simulink model "wifiSwitch"  (R2019b)
settings: Solver=FixedStepAuto  StartTime=0.0  StopTime=inf  RelTol=1e-3  EnableMultiTasking=on
libraries: arduinolib x4
settings Model: SILPILModeSetting=veronly  ExtModeTrigDuration=2  Creator=lucciffer  LastModifiedBy=lucciffer
settings OptimizationCC: EnhancedBackFolding=on  PassReuseOutputArgsAs=Individual arguments  ZeroExternalMemoryAtStartup=off  ZeroInternalMemoryAtStartup=off  MaxStackSize=64  OptimizeBlockOrder=speed  DifferentSizesBufferReuse=on  OptimizationCustomize=off  EfficientTunableParamExpr=on
settings DebuggingCC: ParameterTunabilityLossMsg=error
settings HardwareCC: ProdBitPerInt=16  ProdBitPerPointer=16  ProdBitPerSizeT=16  ProdBitPerPtrDiffT=16  ProdLargestAtomicFloat=None  ProdWordSize=8  ProdHWDeviceType=Atmel->AVR  UseEmbeddedCoderFeatures=off
settings SFSimCC: MATLABDynamicMemAlloc=off
settings RTWCC: SystemTargetFile=ert.tlc  HardwareBoard=Arduino Mega 2560  TLCOptions=-aInlineSetEventsForThisBaseRateFcn=TLC_FALSE -aSuppressMultiTaskScheduler=TLC_FALSE -aRateBasedStepFcn=1  TemplateMakefile=ert_default_tmf  GenerateReport=on  Toolchain=Arduino AVR  BuildConfiguration=Faster Runs  IncludeHyperlinkInReport=on  LaunchReport=on  GenerateTraceInfo=on  GenerateTraceReport=on  GenerateTraceReportSl=on  GenerateTraceReportSf=on  GenerateTraceReportEml=on
settings CodeAppCC: ForceParamTrailComments=on  IgnoreCustomStorageClasses=off  OperatorAnnotations=on  SimulinkDataObjDesc=on  SFDataObjDesc=on  InsertBlockDesc=on
settings ERTTargetCC: SupportContinuousTime=on  SupportNonInlinedSFcns=on  SupportVariableSizeSignals=on  ExtModeStaticAllocSize=2048

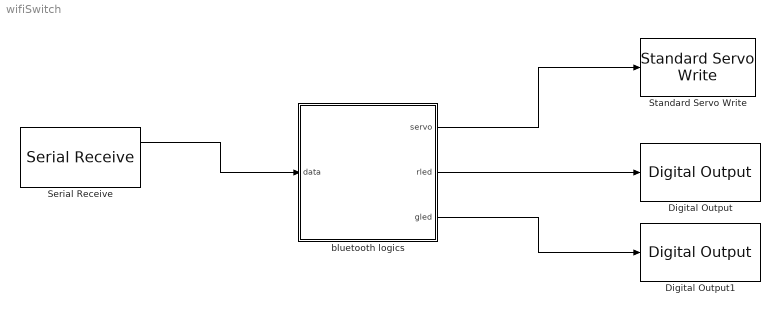
== system wifiSwitch ==
  Digital Output : arduinolib/Digital Output  pinNumber=9  blockPlatform=arduino
  Digital Output1 : arduinolib/Digital Output  pinNumber=10  blockPlatform=arduino
  Serial Receive : arduinolib/Serial Receive  isARMArch=off  portNumber=1  DataType=uint8  Datalength=1  SampleTime=0.1  showOutStatus=on  blockPlatform=arduino
      settings: SourceProductName=Simulink Support Package for Arduino Hardware  SourceProductBaseCode=ARDUINO
  Standard Servo Write : arduinolib/Standard Servo Write  pinNumber=8  ServoIndex=0  blockPlatform=ARDUINO
      settings: SourceProductName=Simulink Support Package for Arduino Hardware
  "bluetooth logics " : Stateflow chart  BlockKeywords=__PRM__SERIALIZED__DATA__:Stateflow Chart,Stateflow Diagram  TreatAsAtomicUnit=on
  wires:
  "bluetooth logics "/2(rled) -> Digital Output/1
  "bluetooth logics "/3(gled) -> Digital Output1/1
  "bluetooth logics "/1(servo) -> Standard Servo Write/1
  Serial Receive/1 -> "bluetooth logics "/1(data)

== stateflow chart wifiSwitch/bluetooth logics  ==
  state ontrans
    servo=110;
    gled=1;
    rled=0;
  state on
    servo=135;
    gled=1;
    rled=0;
  state off
    servo=135;
    gled=0;
    rled=1;
  state offtrans
    servo=110;
    gled=0;
    rled=1;
  on -> ontrans [order 1] : [data=='0']
  ontrans -> on : {after(200,msec)}
  (default) -> on
  off -> on : {after(200,msec)}
  on -> offtrans [order 2] : [data=='1']
  offtrans -> off : {after(200,msec)}
  data: data input; servo output; rled output; gled output
